simulink model "CarSpeedControllerTest1"  (R2023b)
settings: Solver=VariableStepAuto  StartTime=0.0  StopTime=600  RelTol=1e-3
libraries: slpidlib x2
settings Model: Creator=fiona  LastModifiedBy=fiona

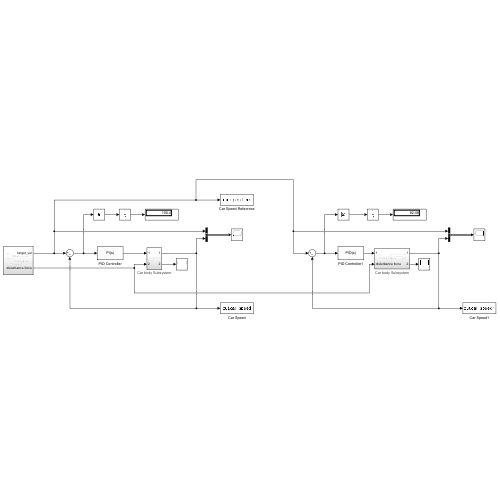
[thumbnail: Simulink's stored preview of the top-level diagram]
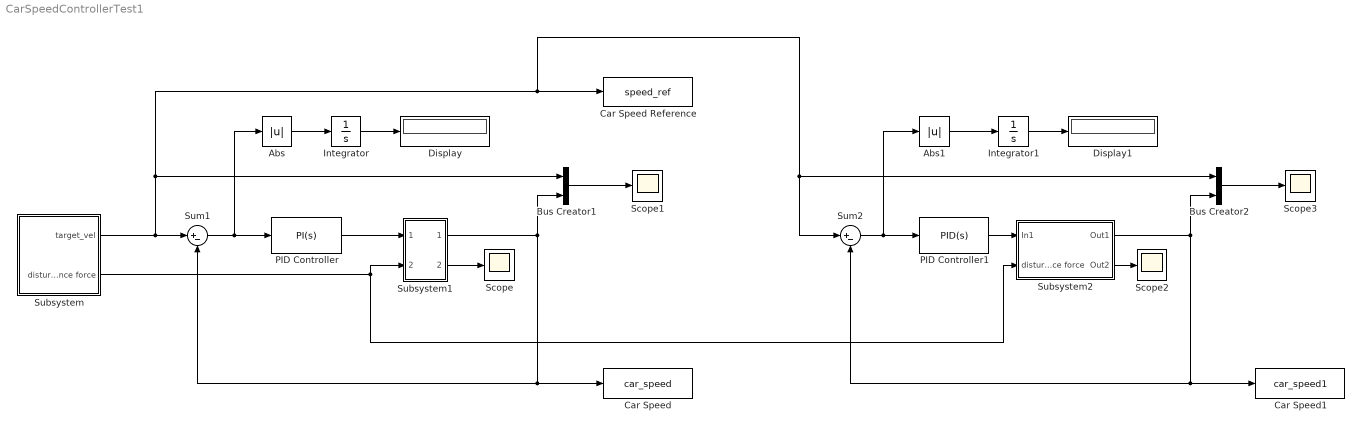
== system CarSpeedControllerTest1 ==
  Abs : Abs  SaturateOnIntegerOverflow=off
  Abs1 : Abs  SaturateOnIntegerOverflow=off
  Bus Creator1 : BusCreator  Inputs=2
  Bus Creator2 : BusCreator  Inputs=2
  Car Speed : ToWorkspace  VariableName=car_speed  SaveFormat=Timeseries  SampleTime=-1
  Car Speed Reference : ToWorkspace  VariableName=speed_ref  SaveFormat=Timeseries  SampleTime=-1
  Car Speed1 : ToWorkspace  VariableName=car_speed1  SaveFormat=Timeseries  SampleTime=-1
  Display : Display
  Display1 : Display
  Integrator : Integrator
  Integrator1 : Integrator
  PID Controller : slpidlib/PID Controller  Controller=PI  Form=Parallel  TimeDomain=Continuous-time  UseExternalTs=off  SampleTime=-1  IntegratorMethod=Forward Euler  FilterMethod=Forward Euler  ControllerParametersSource=internal  P=22.6  I=3.57  UseKiTs=off  D=0  N=100  UseFilter=on  TunerSelectOption=Transfer Function Based (PID Tuner App)  InitialConditionSource=internal  InitialConditionForIntegrator=0  InitialConditionForFilter=0  DifferentiatorICPrevScaledInput=0  ExternalReset=none  TrackingMode=off  Kt=1  LimitOutput=off  SatLimitsSource=internal  UpperSaturationLimit=inf  LowerSaturationLimit=-inf  LinearizeAsGain=on  AntiWindupMode=none  Kb=1  LimitIntegrator=off  UpperIntegratorSaturationLimit=inf  LowerIntegratorSaturationLimit=-inf  POutMin=[]  POutMax=[]  IOutMin=[]  IOutMax=[]  DOutMin=[]  DOutMax=[]  NOutMin=[]  NOutMax=[]  SumOutMin=[]  SumOutMax=[]  SaturationOutMin=[]  SaturationOutMax=[]  PParamMin=[]  PParamMax=[]  IParamMin=[]  IParamMax=[]  DParamMin=[]  DParamMax=[]  NParamMin=[]  NParamMax=[]  KbParamMin=[]  KbParamMax=[]  KtParamMin=[]  KtParamMax=[]  KbOutMin=[]  KbOutMax=[]  KtOutMin=[]  KtOutMax=[]  IntegratorOutMin=[]  IntegratorOutMax=[]  FilterOutMin=[]  FilterOutMax=[]  SumI1OutMin=[]  SumI1OutMax=[]  SumI2OutMin=[]  SumI2OutMax=[]  SumI3OutMin=[]  SumI3OutMax=[]  SumI4OutMin=[]  SumI4OutMax=[]  SumDOutMin=[]  SumDOutMax=[]  DifferentiatorOutMin=[]  DifferentiatorOutMax=[]  FilterDiffOutCoefMin=[]  FilterDiffOutCoefMax=[]  ReciprocalOutMin=[]  ReciprocalOutMax=[]  SumDenOutMin=[]  SumDenOutMax=[]  SumNumOutMin=[]  SumNumOutMax=[]  DivideOutMin=[]  DivideOutMax=[]  UdiffTsProdOutMin=[]  UdiffTsProdOutMax=[]  NTsProdOutMin=[]  NTsProdOutMax=[]  UintegralTsProdOutMin=[]  UintegralTsProdOutMax=[]  UngainTsProdOutMin=[]  UngainTsProdOutMax=[]  ClampingZeroOutDataTypeStr=Inherit: Inherit via back propagation  ClampingZeroOutMin=[]  ClampingZeroOutMax=[]  FilterDenConstantOutDataTypeStr=Inherit: Inherit via back propagation  FilterDenConstantOutMin=[]  FilterDenConstantOutMax=[]  PCopyOutDataTypeStr=Inherit: Inherit via back propagation  PCopyOutMin=[]  PCopyOutMax=[]  NCopyOutDataTypeStr=Inherit: Inherit via back propagation  NCopyOutMin=[]  NCopyOutMax=[]  IntegratorContinuousStateAttributes=''  IntegratorStateMustResolveToSignalObject=off  IntegratorRTWStateStorageClass=Auto  FilterContinuousStateAttributes=''  FilterStateMustResolveToSignalObject=off  FilterRTWStateStorageClass=Auto  ParallelPVariant=InternalParameters  IdealPVariant=Disabled  IVariant=InternalParameters  DVariant=Disabled  IntegratorVariant=Continuous  SatVariant=Disabled  AWVariant=Passthrough  PCopyVariant=Disabled  TRVariant=Disabled  FdbkBlocksVariant=Forward  IdealPFdbkVariant=Disabled  SatFdbkVariant=Disabled  DerivativeFilterVariant=Disabled  NVariant=Disabled  NCopyVariant=Disabled_SignalSpec  FilterICVariant=Disabled  IntegratorICVariant=InternalICs  ExternalResetVariant=Disabled  TRSumVariant=Passthrough  SumFdbkVariant=Disabled  SumVariant=Sum_PI  TsampFilterVariant=InternalTs  TsampNgainVariant=Passthrough  TsampIntegralVariant=Disabled_SignalSpec  ExternalSaturationOutDataTypeStr=Inherit: Same as second input
  PID Controller1 : slpidlib/PID Controller  Controller=PID  Form=Parallel  TimeDomain=Continuous-time  UseExternalTs=off  SampleTime=-1  IntegratorMethod=Forward Euler  FilterMethod=Forward Euler  ControllerParametersSource=internal  P=37  I=0.964  UseKiTs=off  D=10.9  N=2.5  UseFilter=on  TunerSelectOption=Transfer Function Based (PID Tuner App)  InitialConditionSource=internal  InitialConditionForIntegrator=0  InitialConditionForFilter=0  DifferentiatorICPrevScaledInput=0  ExternalReset=none  TrackingMode=off  Kt=1  LimitOutput=off  SatLimitsSource=internal  UpperSaturationLimit=inf  LowerSaturationLimit=-inf  LinearizeAsGain=on  AntiWindupMode=none  Kb=1  LimitIntegrator=off  UpperIntegratorSaturationLimit=inf  LowerIntegratorSaturationLimit=-inf  POutMin=[]  POutMax=[]  IOutMin=[]  IOutMax=[]  DOutMin=[]  DOutMax=[]  NOutMin=[]  NOutMax=[]  SumOutMin=[]  SumOutMax=[]  SaturationOutMin=[]  SaturationOutMax=[]  PParamMin=[]  PParamMax=[]  IParamMin=[]  IParamMax=[]  DParamMin=[]  DParamMax=[]  NParamMin=[]  NParamMax=[]  KbParamMin=[]  KbParamMax=[]  KtParamMin=[]  KtParamMax=[]  KbOutMin=[]  KbOutMax=[]  KtOutMin=[]  KtOutMax=[]  IntegratorOutMin=[]  IntegratorOutMax=[]  FilterOutMin=[]  FilterOutMax=[]  SumI1OutMin=[]  SumI1OutMax=[]  SumI2OutMin=[]  SumI2OutMax=[]  SumI3OutMin=[]  SumI3OutMax=[]  SumI4OutMin=[]  SumI4OutMax=[]  SumDOutMin=[]  SumDOutMax=[]  DifferentiatorOutMin=[]  DifferentiatorOutMax=[]  FilterDiffOutCoefMin=[]  FilterDiffOutCoefMax=[]  ReciprocalOutMin=[]  ReciprocalOutMax=[]  SumDenOutMin=[]  SumDenOutMax=[]  SumNumOutMin=[]  SumNumOutMax=[]  DivideOutMin=[]  DivideOutMax=[]  UdiffTsProdOutMin=[]  UdiffTsProdOutMax=[]  NTsProdOutMin=[]  NTsProdOutMax=[]  UintegralTsProdOutMin=[]  UintegralTsProdOutMax=[]  UngainTsProdOutMin=[]  UngainTsProdOutMax=[]  ClampingZeroOutDataTypeStr=Inherit: Inherit via back propagation  ClampingZeroOutMin=[]  ClampingZeroOutMax=[]  FilterDenConstantOutDataTypeStr=Inherit: Inherit via back propagation  FilterDenConstantOutMin=[]  FilterDenConstantOutMax=[]  PCopyOutDataTypeStr=Inherit: Inherit via back propagation  PCopyOutMin=[]  PCopyOutMax=[]  NCopyOutDataTypeStr=Inherit: Inherit via back propagation  NCopyOutMin=[]  NCopyOutMax=[]  IntegratorContinuousStateAttributes=''  IntegratorStateMustResolveToSignalObject=off  IntegratorRTWStateStorageClass=Auto  FilterContinuousStateAttributes=''  FilterStateMustResolveToSignalObject=off  FilterRTWStateStorageClass=Auto  ParallelPVariant=InternalParameters  IdealPVariant=Disabled  IVariant=InternalParameters  DVariant=InternalParameters  IntegratorVariant=Continuous  SatVariant=Disabled  AWVariant=Passthrough  PCopyVariant=Disabled  TRVariant=Disabled  FdbkBlocksVariant=Forward  IdealPFdbkVariant=Disabled  SatFdbkVariant=Disabled  DerivativeFilterVariant=ContFilter  NVariant=InternalParameters  NCopyVariant=Disabled  FilterICVariant=InternalICsFilter  IntegratorICVariant=InternalICs  ExternalResetVariant=Disabled  TRSumVariant=Passthrough  SumFdbkVariant=Disabled  SumVariant=Sum_PID  TsampFilterVariant=InternalTs  TsampNgainVariant=Passthrough  TsampIntegralVariant=Disabled_SignalSpec  ExternalSaturationOutDataTypeStr=Inherit: Same as second input
  Scope{,1..3} (4 alike) : Scope
  Subsystem : Subsystem
  Subsystem1 : Subsystem
      settings: AttributesFormatString=Car body Subsystem
  Subsystem2 : Subsystem
      settings: AttributesFormatString=Car body Subsystem
  Sum1 : Sum  Inputs=|+-
  Sum2 : Sum  Inputs=|+-
  wires:
  Subsystem1/1(Out1) -> Sum1/2, Car Speed/1, Bus Creator1/2
  Bus Creator1/1 -> Scope1/1
  Subsystem1/2(Out2) -> Scope/1
  Subsystem2/1(Out1) -> Bus Creator2/2, Sum2/2, Car Speed1/1
  Bus Creator2/1 -> Scope3/1
  PID Controller/1 -> Subsystem1/1(In1)
  Sum1/1 -> Abs/1, PID Controller/1
  Abs/1 -> Integrator/1
  Integrator/1 -> Display/1
  Integrator1/1 -> Display1/1
  Abs1/1 -> Integrator1/1
  Sum2/1 -> PID Controller1/1, Abs1/1
  Subsystem/1(target_vel) -> Sum2/1, Bus Creator2/1, Car Speed Reference/1, Bus Creator1/1, Sum1/1
  Subsystem/2(disturbance force) -> Subsystem2/2(disturbance force), Subsystem1/2(In2)
  PID Controller1/1 -> Subsystem2/1(In1)
  Subsystem2/2(Out2) -> Scope2/1

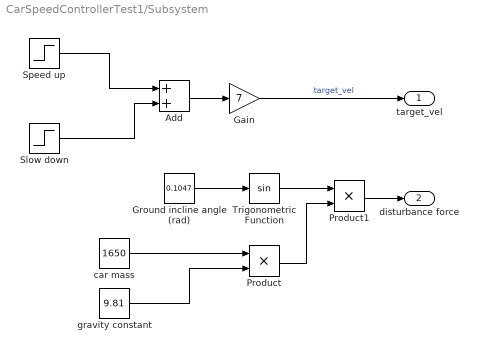
== system CarSpeedControllerTest1/Subsystem ==
  Add : Sum
  Gain : Gain  Gain=7
  Ground incline angle (rad) : Constant  Value=0.1047
  Product : Product
  Product1 : Product
  Slow down : Step  Time=300  Before=3  After=2  SampleTime=0
  Speed up : Step  Time=50  Before=1  After=3  SampleTime=0
  Trigonometric Function : Trigonometry
  car mass : Constant  Value=1650
  gravity constant : Constant  Value=9.81
  target_vel : Outport
  disturbance force : Outport  Port=2
  wires:
  car mass/1 -> Product/1
  Product/1 -> Product1/2
  Ground incline angle (rad)/1 -> Trigonometric Function/1
  Trigonometric Function/1 -> Product1/1
  Add/1 -> Gain/1
  gravity constant/1 -> Product/2
  Slow down/1 -> Add/2
  Speed up/1 -> Add/1
  Gain/1 -> target_vel/1  "target_vel"
  Product1/1 -> disturbance force/1

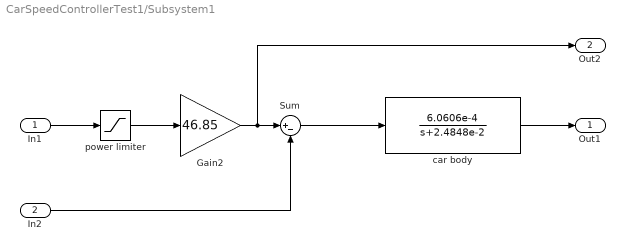
== system CarSpeedControllerTest1/Subsystem1 ==
  In1 : Inport
  In2 : Inport  Port=2
  Gain2 : Gain  Gain=46.85
  Sum : Sum  Inputs=|+-
  car body : TransferFcn  Numerator=[6.0606e-4]  Denominator=[1 2.4848e-2]  ContinuousStateAttributes='position'
  power limiter : Saturate  UpperLimit=1921  LowerLimit=-1921
  Out1 : Outport
  Out2 : Outport  Port=2
  wires:
  Sum/1 -> car body/1
  In1/1 -> power limiter/1
  car body/1 -> Out1/1
  In2/1 -> Sum/2
  power limiter/1 -> Gain2/1
  Gain2/1 -> Out2/1, Sum/1

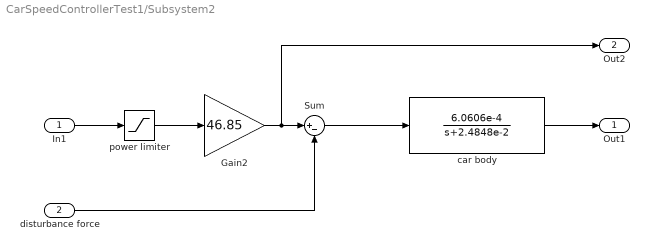
== system CarSpeedControllerTest1/Subsystem2 ==
  In1 : Inport
  disturbance force : Inport  Port=2
  Gain2 : Gain  Gain=46.85
  Sum : Sum  Inputs=|+-
  car body : TransferFcn  Numerator=[6.0606e-4]  Denominator=[1 2.4848e-2]  ContinuousStateAttributes='position'
  power limiter : Saturate  UpperLimit=1921  LowerLimit=-1921
  Out1 : Outport
  Out2 : Outport  Port=2
  wires:
  Sum/1 -> car body/1
  In1/1 -> power limiter/1
  car body/1 -> Out1/1
  disturbance force/1 -> Sum/2
  power limiter/1 -> Gain2/1
  Gain2/1 -> Out2/1, Sum/1
